simulink model "motor_model"  (R2022a)
settings: Solver=VariableStepAuto  StartTime=0.0  StopTime=2  FixedStep=0.001  RelTol=1e-3
values from neighbouring files (symbols this model uses):
  C_csd_den = C_csd.den{:}    [main.m]
  C_csd_num = C_csd.num{:}    [main.m]
  den_c_bench = C_other.Denominator{:}    [main.m]
  den_c_bench_wi = den_c_bench(1:end-1)    [main.m]
  den_si = C_shapeit_manually.den{:}    [main.m]
  den_sys = sys.den{:}    [main.m]
  den_sys_bench = sys.den{:}    [main.m]
  Kd = pid_val.Kd    [main.m]
  Ki = pid_val.Ki    [main.m]
  Kp = pid_val.Kp    [main.m]
  N = 1/pid_val.Tf    [main.m]
  num_c_bench = C_other.Numerator{:}    [main.m]
  num_c_bench_wi = num_c_bench    [main.m]
  num_si = C_shapeit_manually.num{:}    [main.m]
  num_sys = sys.num{:}    [main.m]
  num_sys_bench = sys.num{:}    [main.m]
libraries: slpidlib x3, simulink x1
settings Model: Creator=michi  LastModifiedBy=michi

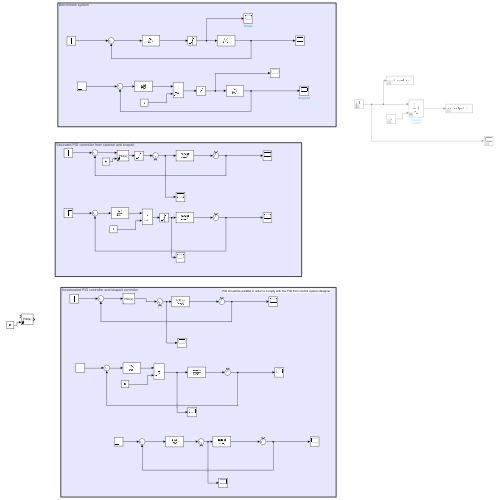
[thumbnail: Simulink's stored preview of the top-level diagram]
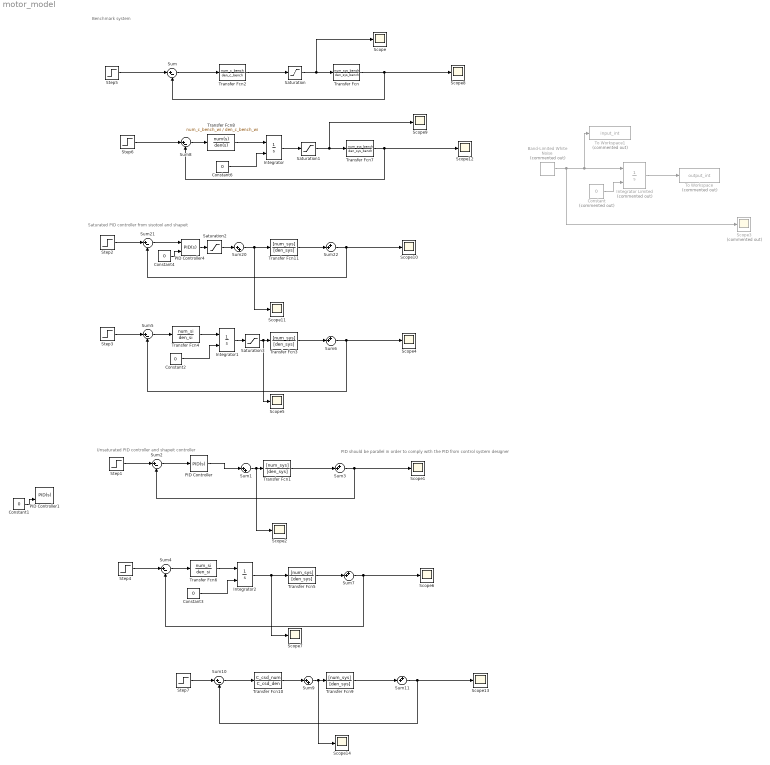
== system motor_model ==
  note: PID should be parallel in order to comply with the PID from control system designer
  note: Unsaturated PID controller and shapeit controller
  note: Saturated PID controller from sisotool and shapeit
  note: Benchmark system
  Band-Limited White Noise : simulink/Sources/Band-Limited White Noise  Commented=on  Cov=[1]  Ts=0.001  seed=[23341]
  Constant : Constant  Commented=on  Value=0
  Constant{1..4,6} (5 alike) : Constant  Value=0
  Integrator : Integrator  ExternalReset=rising  UpperSaturationLimit=3  LowerSaturationLimit=-3
  Integrator Limited : Integrator  Commented=on  ExternalReset=rising  LimitOutput=on  UpperSaturationLimit=3  LowerSaturationLimit=-3
  Integrator1 : Integrator  ExternalReset=rising  UpperSaturationLimit=3  LowerSaturationLimit=-3
  Integrator2 : Integrator  ExternalReset=rising  UpperSaturationLimit=3  LowerSaturationLimit=-3
  PID Controller : slpidlib/PID Controller  Controller=PID  Form=Parallel  TimeDomain=Continuous-time  UseExternalTs=off  SampleTime=-1  IntegratorMethod=Forward Euler  FilterMethod=Forward Euler  ControllerParametersSource=internal  P=Kp  I=Ki  UseKiTs=off  D=Kd  N=N  UseFilter=on  TunerSelectOption=Transfer Function Based (PID Tuner App)  InitialConditionSource=internal  InitialConditionForIntegrator=0  InitialConditionForFilter=0  DifferentiatorICPrevScaledInput=0  ExternalReset=none  TrackingMode=off  Kt=1  LimitOutput=off  SatLimitsSource=internal  UpperSaturationLimit=inf  LowerSaturationLimit=-inf  LinearizeAsGain=on  AntiWindupMode=none  Kb=1  POutMin=[]  POutMax=[]  IOutMin=[]  IOutMax=[]  DOutMin=[]  DOutMax=[]  NOutMin=[]  NOutMax=[]  SumOutMin=[]  SumOutMax=[]  SaturationOutMin=[]  SaturationOutMax=[]  PParamMin=[]  PParamMax=[]  IParamMin=[]  IParamMax=[]  DParamMin=[]  DParamMax=[]  NParamMin=[]  NParamMax=[]  KbParamMin=[]  KbParamMax=[]  KtParamMin=[]  KtParamMax=[]  KbOutMin=[]  KbOutMax=[]  KtOutMin=[]  KtOutMax=[]  IntegratorOutMin=[]  IntegratorOutMax=[]  FilterOutMin=[]  FilterOutMax=[]  SumI1OutMin=[]  SumI1OutMax=[]  SumI2OutMin=[]  SumI2OutMax=[]  SumI3OutMin=[]  SumI3OutMax=[]  SumI4OutMin=[]  SumI4OutMax=[]  SumDOutMin=[]  SumDOutMax=[]  DifferentiatorOutMin=[]  DifferentiatorOutMax=[]  FilterDiffOutCoefMin=[]  FilterDiffOutCoefMax=[]  ReciprocalOutMin=[]  ReciprocalOutMax=[]  SumDenOutMin=[]  SumDenOutMax=[]  SumNumOutMin=[]  SumNumOutMax=[]  DivideOutMin=[]  DivideOutMax=[]  UdiffTsProdOutMin=[]  UdiffTsProdOutMax=[]  NTsProdOutMin=[]  NTsProdOutMax=[]  UintegralTsProdOutMin=[]  UintegralTsProdOutMax=[]  UngainTsProdOutMin=[]  UngainTsProdOutMax=[]  IntegratorContinuousStateAttributes=''  IntegratorStateMustResolveToSignalObject=off  IntegratorRTWStateStorageClass=Auto  FilterContinuousStateAttributes=''  FilterStateMustResolveToSignalObject=off  FilterRTWStateStorageClass=Auto  ParallelPVariant=InternalParameters  IdealPVariant=Disabled  IVariant=InternalParameters  DVariant=InternalParameters  IntegratorVariant=Continuous  SatVariant=Disabled  AWVariant=Passthrough  PCopyVariant=Disabled  TRVariant=Disabled  FdbkBlocksVariant=Forward  IdealPFdbkVariant=Disabled  SatFdbkVariant=Disabled  DerivativeFilterVariant=ContFilter  NVariant=InternalParameters  NCopyVariant=Disabled  FilterICVariant=InternalICsFilter  IntegratorICVariant=InternalICs  ExternalResetVariant=Disabled  TRSumVariant=Passthrough  SumFdbkVariant=Disabled  SumVariant=Sum_PID  TsampFilterVariant=InternalTs  TsampNgainVariant=Passthrough  TsampIntegralVariant=Passthrough  ExternalSaturationOutDataTypeStr=Inherit: Same as second input  aMode=0
  PID Controller1 : slpidlib/PID Controller  Controller=PID  Form=Ideal  TimeDomain=Continuous-time  UseExternalTs=off  SampleTime=-1  IntegratorMethod=Forward Euler  FilterMethod=Forward Euler  ControllerParametersSource=internal  P=Kp  I=Ki  UseKiTs=off  D=Kd  N=N  UseFilter=on  TunerSelectOption=Transfer Function Based (PID Tuner App)  InitialConditionSource=internal  InitialConditionForIntegrator=0  InitialConditionForFilter=0  DifferentiatorICPrevScaledInput=0  ExternalReset=rising  TrackingMode=off  Kt=1  LimitOutput=off  SatLimitsSource=internal  UpperSaturationLimit=inf  LowerSaturationLimit=-inf  LinearizeAsGain=on  AntiWindupMode=none  Kb=1  POutMin=[]  POutMax=[]  IOutMin=[]  IOutMax=[]  DOutMin=[]  DOutMax=[]  NOutMin=[]  NOutMax=[]  SumOutMin=[]  SumOutMax=[]  SaturationOutMin=[]  SaturationOutMax=[]  PParamMin=[]  PParamMax=[]  IParamMin=[]  IParamMax=[]  DParamMin=[]  DParamMax=[]  NParamMin=[]  NParamMax=[]  KbParamMin=[]  KbParamMax=[]  KtParamMin=[]  KtParamMax=[]  KbOutMin=[]  KbOutMax=[]  KtOutMin=[]  KtOutMax=[]  IntegratorOutMin=[]  IntegratorOutMax=[]  FilterOutMin=[]  FilterOutMax=[]  SumI1OutMin=[]  SumI1OutMax=[]  SumI2OutMin=[]  SumI2OutMax=[]  SumI3OutMin=[]  SumI3OutMax=[]  SumI4OutMin=[]  SumI4OutMax=[]  SumDOutMin=[]  SumDOutMax=[]  DifferentiatorOutMin=[]  DifferentiatorOutMax=[]  FilterDiffOutCoefMin=[]  FilterDiffOutCoefMax=[]  ReciprocalOutMin=[]  ReciprocalOutMax=[]  SumDenOutMin=[]  SumDenOutMax=[]  SumNumOutMin=[]  SumNumOutMax=[]  DivideOutMin=[]  DivideOutMax=[]  UdiffTsProdOutMin=[]  UdiffTsProdOutMax=[]  NTsProdOutMin=[]  NTsProdOutMax=[]  UintegralTsProdOutMin=[]  UintegralTsProdOutMax=[]  UngainTsProdOutMin=[]  UngainTsProdOutMax=[]  IntegratorContinuousStateAttributes=''  IntegratorStateMustResolveToSignalObject=off  IntegratorRTWStateStorageClass=Auto  FilterContinuousStateAttributes=''  FilterStateMustResolveToSignalObject=off  FilterRTWStateStorageClass=Auto  ParallelPVariant=Passthrough  IdealPVariant=InternalParameters  IVariant=InternalParameters  DVariant=InternalParameters  IntegratorVariant=Continuous  SatVariant=Disabled  AWVariant=Passthrough  PCopyVariant=Disabled  TRVariant=Disabled  FdbkBlocksVariant=Forward  IdealPFdbkVariant=Disabled  SatFdbkVariant=Disabled  DerivativeFilterVariant=ContFilter  NVariant=InternalParameters  NCopyVariant=Disabled  FilterICVariant=InternalICsFilter  IntegratorICVariant=InternalICs  ExternalResetVariant=ExternalReset  TRSumVariant=Passthrough  SumFdbkVariant=Disabled  SumVariant=Sum_PID  TsampFilterVariant=InternalTs  TsampNgainVariant=Passthrough  TsampIntegralVariant=Passthrough  ExternalSaturationOutDataTypeStr=Inherit: Same as second input  aMode=0
  PID Controller4 : slpidlib/PID Controller  Controller=PID  Form=Parallel  TimeDomain=Continuous-time  UseExternalTs=off  SampleTime=-1  IntegratorMethod=Forward Euler  FilterMethod=Forward Euler  ControllerParametersSource=internal  P=Kp  I=Ki  UseKiTs=off  D=Kd  N=N  UseFilter=on  TunerSelectOption=Transfer Function Based (PID Tuner App)  InitialConditionSource=internal  InitialConditionForIntegrator=0  InitialConditionForFilter=0  DifferentiatorICPrevScaledInput=0  ExternalReset=rising  TrackingMode=off  Kt=1  LimitOutput=off  SatLimitsSource=internal  UpperSaturationLimit=inf  LowerSaturationLimit=-inf  LinearizeAsGain=on  AntiWindupMode=none  Kb=1  POutMin=[]  POutMax=[]  IOutMin=[]  IOutMax=[]  DOutMin=[]  DOutMax=[]  NOutMin=[]  NOutMax=[]  SumOutMin=[]  SumOutMax=[]  SaturationOutMin=[]  SaturationOutMax=[]  PParamMin=[]  PParamMax=[]  IParamMin=[]  IParamMax=[]  DParamMin=[]  DParamMax=[]  NParamMin=[]  NParamMax=[]  KbParamMin=[]  KbParamMax=[]  KtParamMin=[]  KtParamMax=[]  KbOutMin=[]  KbOutMax=[]  KtOutMin=[]  KtOutMax=[]  IntegratorOutMin=[]  IntegratorOutMax=[]  FilterOutMin=[]  FilterOutMax=[]  SumI1OutMin=[]  SumI1OutMax=[]  SumI2OutMin=[]  SumI2OutMax=[]  SumI3OutMin=[]  SumI3OutMax=[]  SumI4OutMin=[]  SumI4OutMax=[]  SumDOutMin=[]  SumDOutMax=[]  DifferentiatorOutMin=[]  DifferentiatorOutMax=[]  FilterDiffOutCoefMin=[]  FilterDiffOutCoefMax=[]  ReciprocalOutMin=[]  ReciprocalOutMax=[]  SumDenOutMin=[]  SumDenOutMax=[]  SumNumOutMin=[]  SumNumOutMax=[]  DivideOutMin=[]  DivideOutMax=[]  UdiffTsProdOutMin=[]  UdiffTsProdOutMax=[]  NTsProdOutMin=[]  NTsProdOutMax=[]  UintegralTsProdOutMin=[]  UintegralTsProdOutMax=[]  UngainTsProdOutMin=[]  UngainTsProdOutMax=[]  IntegratorContinuousStateAttributes=''  IntegratorStateMustResolveToSignalObject=off  IntegratorRTWStateStorageClass=Auto  FilterContinuousStateAttributes=''  FilterStateMustResolveToSignalObject=off  FilterRTWStateStorageClass=Auto  ParallelPVariant=InternalParameters  IdealPVariant=Disabled  IVariant=InternalParameters  DVariant=InternalParameters  IntegratorVariant=Continuous  SatVariant=Disabled  AWVariant=Passthrough  PCopyVariant=Disabled  TRVariant=Disabled  FdbkBlocksVariant=Forward  IdealPFdbkVariant=Disabled  SatFdbkVariant=Disabled  DerivativeFilterVariant=ContFilter  NVariant=InternalParameters  NCopyVariant=Disabled  FilterICVariant=InternalICsFilter  IntegratorICVariant=InternalICs  ExternalResetVariant=ExternalReset  TRSumVariant=Passthrough  SumFdbkVariant=Disabled  SumVariant=Sum_PID  TsampFilterVariant=InternalTs  TsampNgainVariant=Passthrough  TsampIntegralVariant=Passthrough  ExternalSaturationOutDataTypeStr=Inherit: Same as second input  aMode=0
  Saturation{,1..3} (4 alike) : Saturate  UpperLimit=3  LowerLimit=-3
  Scope{,1..2,4..14} (14 alike) : Scope
  Scope3 : Scope  Commented=on
  Step{1..4,7} (5 alike) : Step  After=0.01  SampleTime=0
  Step5 : Step  After=0.008  SampleTime=0
  Step6 : Step  After=0.008  SampleTime=0
  Sum{,2,4..5,8,10,21} (7 alike) : Sum  Inputs=|+-
  Sum1 : Sum  Inputs=|++
  Sum{3,6..7,11,22} (5 alike) : Sum  Inputs=++|
  Sum20 : Sum  Inputs=|++
  Sum9 : Sum  Inputs=|++
  To Workspace : ToWorkspace  Commented=on  VariableName=output_int  SampleTime=-1
  To Workspace1 : ToWorkspace  Commented=on  VariableName=input_int  SampleTime=-1
  Transfer Fcn : TransferFcn  Numerator=num_sys_bench  Denominator=den_sys_bench
  Transfer Fcn{1,3,5,9,11} (5 alike) : TransferFcn  Numerator=[num_sys]  Denominator=[den_sys]
  Transfer Fcn10 : TransferFcn  Numerator=C_csd_num  Denominator=C_csd_den
  Transfer Fcn2 : TransferFcn  Numerator=num_c_bench  Denominator=den_c_bench
  Transfer Fcn4 : TransferFcn  Numerator=num_si  Denominator=den_si
  Transfer Fcn6 : TransferFcn  Numerator=num_si  Denominator=den_si
  Transfer Fcn7 : TransferFcn  Numerator=num_sys_bench  Denominator=den_sys_bench
  Transfer Fcn8 : TransferFcn  Numerator=num_c_bench_wi  Denominator=den_c_bench_wi
  wires:
  Constant/1 -> Integrator Limited/2
  Band-Limited White Noise/1 -> Scope3/1, To Workspace1/1, Integrator Limited/1
  Integrator Limited/1 -> To Workspace/1
  PID Controller4/1 -> Saturation2/1
  Sum21/1 -> PID Controller4/1
  Transfer Fcn11/1 -> Sum22/2
  Sum20/1 -> Scope11/1, Transfer Fcn11/1
  Constant4/1 -> PID Controller4/2
  Step2/1 -> Sum21/1
  Saturation2/1 -> Sum20/1
  Sum22/1 -> Scope10/1, Sum21/2
  Sum3/1 -> Scope1/1, Sum2/2
  Transfer Fcn1/1 -> Sum3/2
  Step1/1 -> Sum2/1
  Constant1/1 -> PID Controller1/2
  Sum1/1 -> Scope2/1, Transfer Fcn1/1
  Step5/1 -> Sum/1
  Transfer Fcn/1 -> Scope8/1, Sum/2
  Sum/1 -> Transfer Fcn2/1
  Saturation/1 -> Scope/1, Transfer Fcn/1
  Step3/1 -> Sum5/1
  Sum6/1 -> Scope4/1, Sum5/2
  Transfer Fcn3/1 -> Sum6/2
  Transfer Fcn4/1 -> Integrator1/1
  Sum5/1 -> Transfer Fcn4/1
  Sum4/1 -> Transfer Fcn6/1
  Transfer Fcn6/1 -> Integrator2/1
  Step4/1 -> Sum4/1
  Transfer Fcn5/1 -> Sum7/2
  Integrator2/1 -> Scope7/1, Transfer Fcn5/1
  Sum7/1 -> Scope6/1, Sum4/2
  Transfer Fcn2/1 -> Saturation/1
  Transfer Fcn7/1 -> Scope12/1, Sum8/2
  Saturation1/1 -> Scope9/1, Transfer Fcn7/1
  Step6/1 -> Sum8/1
  Sum8/1 -> Transfer Fcn8/1
  Transfer Fcn8/1 -> Integrator/1
  Integrator/1 -> Saturation1/1
  Constant6/1 -> Integrator/2
  Constant2/1 -> Integrator1/2
  Constant3/1 -> Integrator2/2
  Integrator1/1 -> Saturation3/1
  Saturation3/1 -> Scope5/1, Transfer Fcn3/1
  Step7/1 -> Sum10/1
  Transfer Fcn9/1 -> Sum11/2
  Sum9/1 -> Scope14/1, Transfer Fcn9/1
  Sum11/1 -> Scope13/1, Sum10/2
  Sum10/1 -> Transfer Fcn10/1
  Transfer Fcn10/1 -> Sum9/1
  Sum2/1 -> PID Controller/1
  PID Controller/1 -> Sum1/1
